simulink model "Xe_chay_diem_target_khong_huong_theta"  (R2021b)
settings: Solver=VariableStepAuto  StartTime=0.0  StopTime=10  RelTol=1e-3
libraries: simulink_extras x1
settings Model: Creator=HL_1810  LastModifiedBy=ASUS

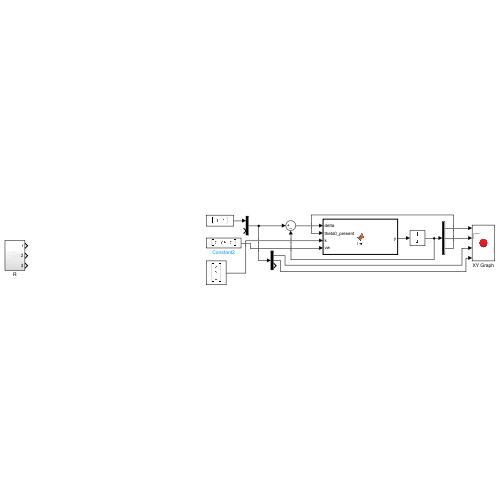
[thumbnail: Simulink's stored preview of the top-level diagram]
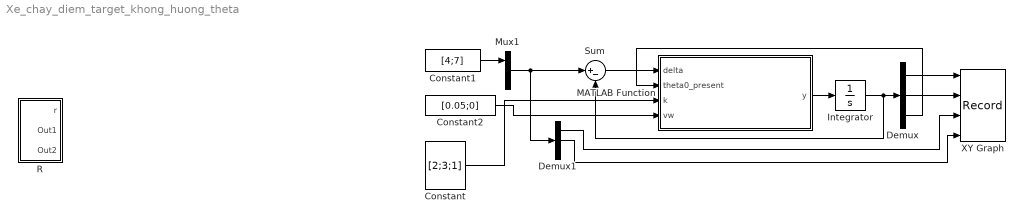
== system Xe_chay_diem_target_khong_huong_theta ==
  Constant : Constant  Value=[2;3;1]  VectorParams1D=off
  Constant1 : Constant  Value=[4;7]
  Constant2 : Constant  Value=[0.05;0]
  Demux : Demux  Outputs=3
  Demux1 : Demux  Outputs=3
  Integrator : Integrator  InitialCondition=[2;2;pi/4]
  MATLAB Function : MATLAB Function  TreatAsAtomicUnit=on
  Mux1 : Mux  Inputs=2
  R : Subsystem
  Sum : Sum  Inputs=|+-
  XY Graph : Record  FileSettingsInternal="{\"entries\":[{\"content\":{\"excelSettings\":{\"content\":{},\"type\":\"Streamout.ExcelSettings\"}},\"type\":\"Streamout.FileSettingStorage\",\"uuid\":\"327fa276-bddc-4a30-a90d-6ce471a90d6d\"}],\"packageUris\":[\"http://schema.mathworks.com/mf0/streamout_blocks/R2020a\"],\"version\":\"1.0\"}"  Layout=[1 1]  SignalsInternal="{\"entries\":[{\"content\":{\"signals\":[{\"content\":{\"blockPath\":[\"Xe_chay_diem_target_khong_huong_theta/XY Graph\"],\"channel\":[],\"dimensions\":[1],\"domain\":\"Xe_chay_diem_target_khong_huong_theta/XY Graph\",\"lineColor\":\"#64d413\",\"plots\":[1],\"port\":1,\"sid\":[],\"signalID\":4977,\"signalName\":\"X xe\"},\"type\":\"RecordBlkView.Signal\",\"uuid\":\"2c9c0063-3d7d-4505-bbcb-27bf7b98b8ce\"},{\"content\":{\"blockPath\":[\"Xe_chay_diem_target_khong_huong_theta/XY Graph\"],\"channel\":[],\"dimensions\":[1],\"domain\":\"Xe_chay_diem_target_khong_huong_theta/XY Graph\",\"lineColor\":\"#ff13a6\",\"plots\":[1],\"port\":2,\"sid\":[],\"signalID\":4980,\"signalName\":\"Y xe\"},\"type\":\"RecordBlkView.Signal\",\"uuid\":\"548a605f-d045-4ffa-a3b2-29941a8de17a\"},{\"content\":{\"blockPath\":[\"Xe_chay_diem_target_khong_huong_theta/XY Graph\"],\"channel\":[],\"dimensions\":[1],\"domain\":\"Xe_chay_diem_target_khong_huong_theta/XY Graph\",\"lineColor\":\"#fe330a\",\"plots\":[1,2],\"port\":3,\"sid\":[],\"signalID\":4983,\"signalName\":\"X target\"},\"type\":\"RecordBlkView.Signal\",\"uuid\":\"36cc6664-c03e-432c-a1af-102d63e8dfa8\"},{\"content\":{\"blockPath\":[\"Xe_chay_diem_target_khong_huong_theta/XY Graph\"],\"channel\":[],\"dimensions\":[1],\"domain\":\"Xe_chay_diem_target_khong_huong_theta/XY Graph\",\"lineColor\":\"#22b573\",\"plots\":[1,2],\"port\":4,\"sid\":[],\"signalID\":4986,\"signalName\":\"Y target\"},\"type\":\"RecordBlkView.Signal\",\"uuid\":\"ba420748-a3e4-44e7-b2ef-4096040c503d\"}]},\"type\":\"RecordBlkView.InputSignals\",\"uuid\":\"189e08d2-94e0-431e-9bba-9e553e9c646a\"}],\"packageUris\":[\"http://schema.mathworks.com/mf0/streamout_blocks/R2020a\"],\"version\":\"1.0\"}"  VisualizationBindings="{\"xyplotplugin\":{\"info\":[{\"series\":[{\"bindingParametersList\":[{\"parameter\":\"X-Axis\",\"signalID\":4977,\"signalName\":\"X xe\"},{\"parameter\":\"Y-Axis\",\"signalID\":4980,\"signalName\":\"Y xe\"}],\"seriesID\":23154},{\"bindingParametersList\":[{\"parameter\":\"X-Axis\",\"signalID\":4983,\"signalName\":\"X target\"},{\"parameter\":\"Y-Axis\",\"signalID\":4986,\"signalName\":\"Y target\"}],\"seriesID\":43328}],\"subplotID\":1},{\"series\":[{\"bindingParametersList\":[{\"parameter\":\"X-Axis\",\"signalID\":4983,\"signalName\":\"X target\"},{\"parameter\":\"Y-Axis\",\"signalID\":4986,\"signalName\":\"Y target\"}],\"seriesID\":47710}],\"subplotID\":2}]}}"  CompatibilityTag=XY
  wires:
  Demux/2 -> XY Graph/2
  Demux/1 -> XY Graph/1
  Demux/3 -> MATLAB Function/2(theta0_present)
  Constant/1 -> MATLAB Function/3(k)
  MATLAB Function/1(y) -> Integrator/1
  Integrator/1 -> Sum/2, Demux/1
  Sum/1 -> MATLAB Function/1(delta)
  Demux1/1 -> XY Graph/3
  Demux1/2 -> XY Graph/4
  Constant1/1 -> Mux1/1
  Mux1/1 -> Sum/1, Demux1/1
  Constant2/1 -> MATLAB Function/4(vw)

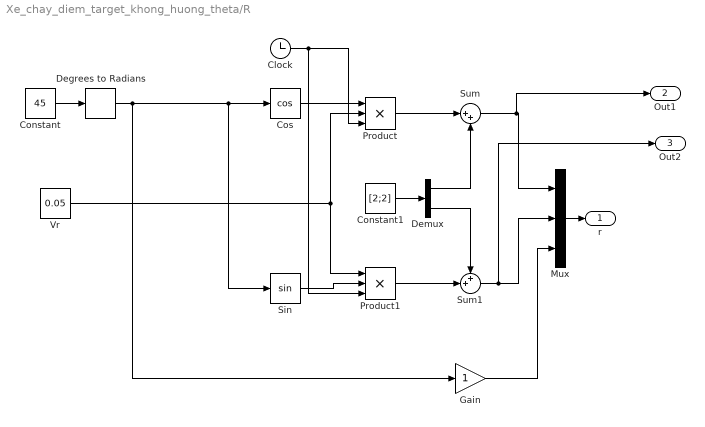
== system Xe_chay_diem_target_khong_huong_theta/R ==
  Clock : Clock
  Constant : Constant  Value=45
  Constant1 : Constant  Value=[2;2]
  Cos : Trigonometry  Operator=cos
  Degrees to Radians : simulink_extras/Transformations/Degrees to Radians
  Demux : Demux  Outputs=2
  Gain : Gain
  Mux : Mux  Inputs=3
  Product : Product  Inputs=3
  Product1 : Product  Inputs=3
  Sin : Trigonometry
  Sum : Sum  Inputs=|++
  Sum1 : Sum  Inputs=++|
  Vr : Constant  Value=0.05
  r : Outport
  Out1 : Outport  Port=2
  Out2 : Outport  Port=3
  wires:
  Sum1/1 -> Out2/1, Mux/2
  Constant1/1 -> Demux/1
  Constant/1 -> Degrees to Radians/1
  Clock/1 -> Product1/3, Product/3
  Cos/1 -> Product/1
  Degrees to Radians/1 -> Gain/1, Sin/1, Cos/1
  Sin/1 -> Product1/2
  Sum/1 -> Out1/1, Mux/1
  Gain/1 -> Mux/3
  Product1/1 -> Sum1/2
  Vr/1 -> Product1/1, Product/2
  Product/1 -> Sum/1
  Demux/2 -> Sum1/1
  Demux/1 -> Sum/2
  Mux/1 -> r/1

== matlab function Xe_chay_diem_target_khong_huong_theta/MATLAB Function ==
  data: delta input; y output; theta0_present input; k input; vw input
function y = fcn(delta,theta0_present,k,vw)
%#codegen
A=[cos(theta0_present)   sin(theta0_present) 0;
    -sin(theta0_present) cos(theta0_present) 0;
    0                    0                    1];
e=A*delta;
V_c=[vw(1)*cos(e(3))+k(1)*e(1);
    vw(2)+k(2)*vw(1)*e(2)+k(3)*vw(1)*sin(e(3))];
Matrix=[cos(theta0_present) 0;
        sin(theta0_present) 0;
        0                   1];
u=Matrix*V_c;
y = u;
